simulink model "basic_spring_mass_damper"  (R2019a)
settings: Solver=VariableStepAuto  StartTime=0.0  StopTime=100  RelTol=1e-3
values from neighbouring files (symbols this model uses):
  A = 3    [trail.m]
  b = 2    [trail.m]
  epsilon = 0.05    [trail.m]
  f_k = 5    [trail.m]
  k = 25    [trail.m]
  M = 4    [Simulation_Script.m]    (also in trail.m = 10; trail2.m)
settings Model: Creator=Lenovo  LastModifiedBy=Lenovo
settings DataIOCC: ReturnWorkspaceOutputs=off
settings DebuggingCC: ArithmeticOperatorsInVariantConditions=warning

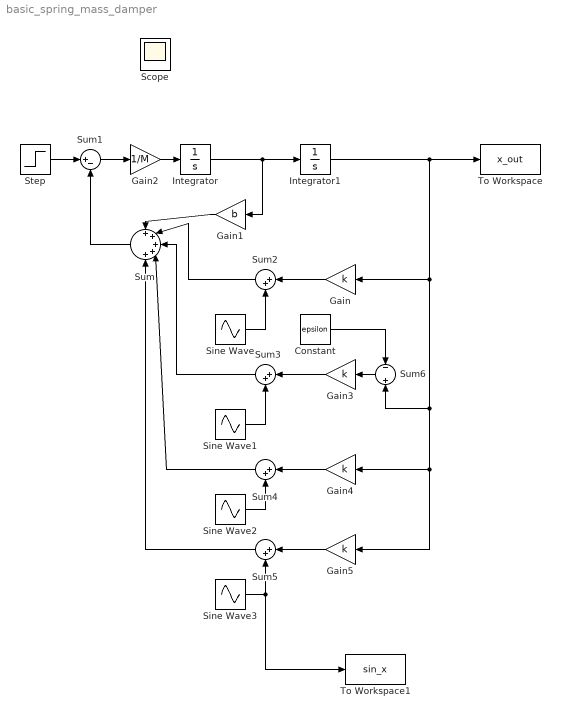
== system basic_spring_mass_damper ==
  Constant : Constant  Value=epsilon
  Gain{,3..5} (4 alike) : Gain  Gain=k
  Gain1 : Gain  Gain=b
  Gain2 : Gain  Gain=1/M
  Integrator : Integrator
  Integrator1 : Integrator
  Sine Wave{,1..3} (4 alike) : Sin  Amplitude=A  Frequency=pi*2*f_k  SampleTime=0.001
  Step : Step  After=0.1  SampleTime=0.001
  Sum : Sum  Inputs=+++++
  Sum1 : Sum  Inputs=|+-
  Sum{2..5} (4 alike) : Sum  Inputs=|++
  Sum6 : Sum  Inputs=-||+
  To Workspace : ToWorkspace  VariableName=x_out  SaveFormat=Timeseries  SampleTime=-1
  To Workspace1 : ToWorkspace  VariableName=sin_x  SaveFormat=Timeseries  SampleTime=-1
  Scope : Scope
  wires:
  Integrator/1 -> Gain1/1, Integrator1/1
  Gain1/1 -> Sum/1
  Sum/1 -> Sum1/2
  Sum1/1 -> Gain2/1
  Step/1 -> Sum1/1
  Gain2/1 -> Integrator/1
  Sum2/1 -> Sum/2
  Gain/1 -> Sum2/1
  Sine Wave/1 -> Sum2/2
  Sum3/1 -> Sum/3
  Gain3/1 -> Sum3/1
  Sine Wave1/1 -> Sum3/2
  Sum4/1 -> Sum/4
  Gain4/1 -> Sum4/1
  Sine Wave2/1 -> Sum4/2
  Gain5/1 -> Sum5/1
  Integrator1/1 -> To Workspace/1, Sum6/2, Gain5/1, Gain4/1, Gain/1
  Sine Wave3/1 -> Sum5/2, To Workspace1/1
  Sum5/1 -> Sum/5
  Sum6/1 -> Gain3/1
  Constant/1 -> Sum6/1
